simulink model "mealy_vending_machine"  (R2020b)
settings: Solver=VariableStepAuto  StartTime=0.0  StopTime=200  RelTol=1e-3
settings Model: Creator=shraddha  LastModifiedBy=shraddha

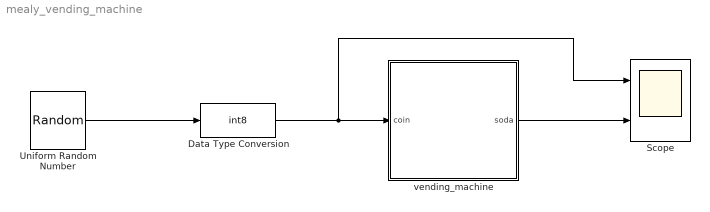
== system mealy_vending_machine ==
  Data Type Conversion : DataTypeConversion  OutDataTypeStr=int8  RndMeth=Nearest
  Scope : Scope  NumInputPorts=2
  Uniform Random Number : UniformRandomNumber  Minimum=0  Maximum=2  Seed=337  SampleTime=10
  vending_machine : Stateflow chart  TreatAsAtomicUnit=on
  wires:
  Uniform Random Number/1 -> Data Type Conversion/1
  Data Type Conversion/1 -> Scope/1, vending_machine/1(coin)
  vending_machine/1(soda) -> Scope/2

== stateflow chart mealy_vending_machine/vending_machine ==
  state got_0
  state got_nickel
  state got_dime
  (default) -> got_0
  got_0 -> got_nickel [order 1] : [coin==1]{soda=0}
  got_nickel -> got_0 [order 1] : [coin==2]{soda=1}
  got_0 -> got_dime [order 2] : [coin==2]{soda=0}
  got_dime -> got_0 [order 2] : [coin==1]{soda=1}
  got_nickel -> got_dime [order 2] : [coin==1]{soda=0}
  got_dime -> got_nickel [order 1] : [coin==2]{soda=1}
  data: coin input; soda output
